simulink library "Desat_Controller_Logic_lib"  (R2018b)
settings: Solver=VariableStepAuto  StartTime=0.0  StopTime=10.0  RelTol=1e-3
undefined symbols (not defined in the file): fswParams
settings Model: Creator=colem  LastModifiedBy=colem

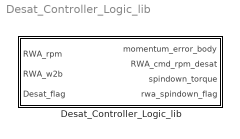
== system Desat_Controller_Logic_lib ==
  Desat_Controller_Logic_lib : Subsystem

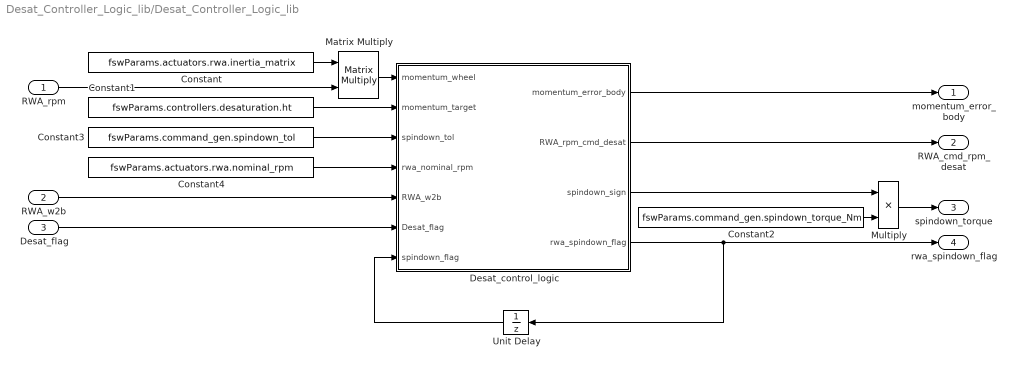
== system Desat_Controller_Logic_lib/Desat_Controller_Logic_lib ==
  RWA_rpm : Inport
  RWA_w2b : Inport  Port=2
  Desat_flag : Inport  Port=3
  Constant : Constant  Value=fswParams.actuators.rwa.inertia_matrix  SampleTime=fswParams.sample_time_s
  Constant1 : Constant  Value=fswParams.controllers.desaturation.ht  SampleTime=fswParams.sample_time_s
  Constant2 : Constant  Value=fswParams.command_gen.spindown_torque_Nm  SampleTime=fswParams.sample_time_s
  Constant3 : Constant  Value=fswParams.command_gen.spindown_tol  SampleTime=fswParams.sample_time_s
  Constant4 : Constant  Value=fswParams.actuators.rwa.nominal_rpm  SampleTime=fswParams.sample_time_s
  Desat_control_logic : MATLAB Function  TreatAsAtomicUnit=on
  Matrix Multiply : Product  Multiplication=Matrix(*)
  Multiply : Product
  Unit Delay : UnitDelay  SampleTime=-1
  momentum_error_body : Outport
  RWA_cmd_rpm_desat : Outport  Port=2
  spindown_torque : Outport  Port=3
  rwa_spindown_flag : Outport  Port=4
  wires:
  Desat_control_logic/1(momentum_error_body) -> momentum_error_body/1
  Desat_control_logic/2(RWA_rpm_cmd_desat) -> RWA_cmd_rpm_desat/1
  Constant/1 -> Matrix Multiply/1
  RWA_w2b/1 -> Desat_control_logic/5(RWA_w2b)
  Desat_control_logic/4(rwa_spindown_flag) -> rwa_spindown_flag/1, Unit Delay/1
  RWA_rpm/1 -> Matrix Multiply/2
  Matrix Multiply/1 -> Desat_control_logic/1(momentum_wheel)
  Constant1/1 -> Desat_control_logic/2(momentum_target)
  Desat_flag/1 -> Desat_control_logic/6(Desat_flag)
  Desat_control_logic/3(spindown_sign) -> Multiply/1
  Multiply/1 -> spindown_torque/1
  Constant2/1 -> Multiply/2
  Unit Delay/1 -> Desat_control_logic/7(spindown_flag)
  Constant3/1 -> Desat_control_logic/3(spindown_tol)
  Constant4/1 -> Desat_control_logic/4(rwa_nominal_rpm)

== matlab function Desat_Controller_Logic_lib/Desat_control_logic ==
  data: momentum_wheel input; momentum_error_body output; momentum_target input; spindown_tol input; rwa_nominal_rpm input; RWA_w2b input; RWA_rpm_cmd_desat output; spindown_sign output; rwa_spindown_flag output; Desat_flag input; spindown_flag input
function [momentum_error_body, RWA_rpm_cmd_desat, spindown_sign, rwa_spindown_flag] ... 
    = desat_control_logic(momentum_wheel, momentum_target, spindown_tol, rwa_nominal_rpm,...
        RWA_w2b, Desat_flag, spindown_flag)

%#codegen

% Author: Cole Morgan
%
% Function to work around the issue with desaturation in the Sidi book. 
% Here, we have more than 3 wheels, so we have a non-trivial nullspace.
% The wheels will eventually get driven to the nullspace while
% desaturating. This checks if they are stuck and need to be commanded in
% "open loop" (not based on a feedback control law) down to their target
% setpoint.



rwa_spindown_flag = 0;

momentum_error_wheel = momentum_wheel - momentum_target;
momentum_error_body  = RWA_w2b*momentum_error_wheel;

spindown_sign = zeros(length(momentum_error_wheel), 1);

tol = 3*0.0012; % based on rpm to momentum for each wheel. ammounts to like 45 rpm I think.

if(Desat_flag)
    % Check to see if there is no excess momentum in the body frame. If there
    % is none, you are in the nullspace issue because you are still in desat
    % mode to be here.
    if (max(abs(momentum_error_body)) < spindown_tol || spindown_flag)

        % The sc bus should still be stable. Therefore, we can send the wheels
        % to another area of the nullspace whereby they store the same amount of angular momentum
        % without changing the total stored momentum of the system, and the bus
        % will remain stable
        RWA_rpm_cmd_desat = rwa_nominal_rpm;
        
        % spin down with a torque opposite the excess momentum of the wheel.
        spindown_sign     = -sign(momentum_error_wheel);
        rwa_spindown_flag = 1;
        return
    end
end

% will likely not reach this point as we will be brought out of desat mode
% at about 1060rpm.
rwa_spindown_flag = 0;

% ensure we have output for variable. Set to zero so it does not interfere.
RWA_rpm_cmd_desat = [0;0;0;0];
end
